simulink model "mathematical_inverted_pendulum_2018"  (R2018a)
settings: Solver=ode5  StartTime=0.0  StopTime=2  FixedStep=10e-6  RelTol=1e-3
values from neighbouring files (symbols this model uses):
  b = 0.1    [inverted_pendulum_parameter.m]
  g = 9.8    [inverted_pendulum_parameter.m]
  I = 0.006    [inverted_pendulum_parameter.m]
  l = 0.3    [inverted_pendulum_parameter.m]
  M = 0.5    [inverted_pendulum_parameter.m]
  m = 0.2    [inverted_pendulum_parameter.m]
settings Model: Creator=Goku  LastModifiedBy=root
settings DataIOCC: ReturnWorkspaceOutputs=on
settings DebuggingCC: InitInArrayFormatMsg=none
settings SFSimCC: SimUseLocalCustomCode=on
settings RTWCC: RTWUseLocalCustomCode=on

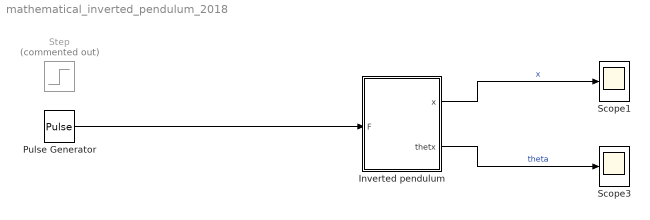
== system mathematical_inverted_pendulum_2018 ==
  Inverted pendulum : Subsystem
  Pulse Generator : DiscretePulseGenerator  PulseType=Time based  Amplitude=1000  Period=10  PulseWidth=0.01
  Scope1 : Scope
  Scope3 : Scope
  Step : Step  Commented=on  Time=0.01  Before=1  After=0  SampleTime=0
  wires:
  Inverted pendulum/1(x) -> Scope1/1  "x"
  Inverted pendulum/2(thetx) -> Scope3/1  "theta"
  Pulse Generator/1 -> Inverted pendulum/1(F)

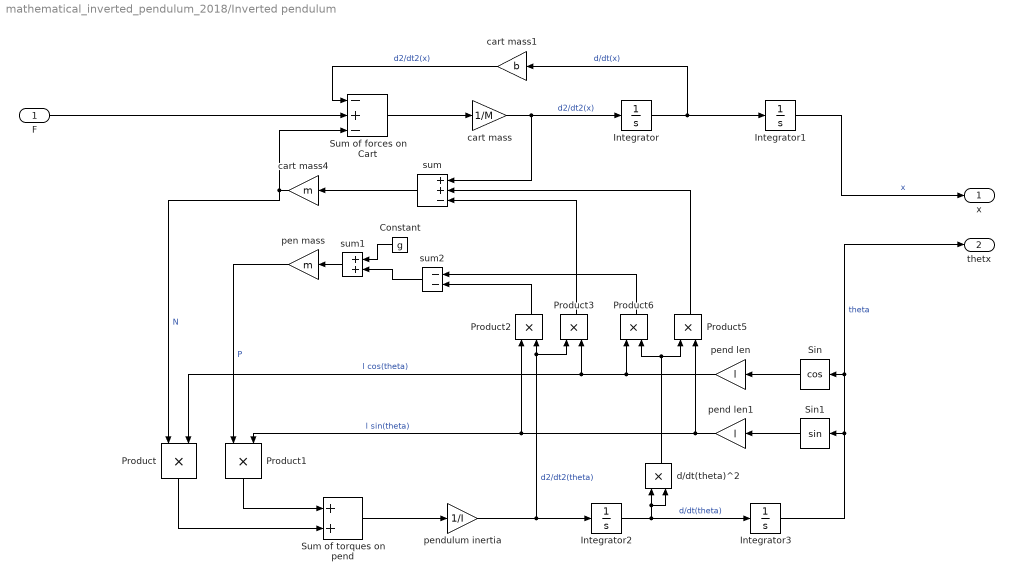
== system mathematical_inverted_pendulum_2018/Inverted pendulum ==
  F : Inport
  Constant : Constant  Value=g
  Integrator{,1..3} (4 alike) : Integrator
  Product{,1..3,5..6} (6 alike) : Product
  Sin : Trigonometry  Operator=cos
  Sin1 : Trigonometry
  Sum of forces on Cart : Sum  Inputs=-+-
  Sum of torques on pend : Sum
  cart mass : Gain  Gain=1/M
  cart mass1 : Gain  Gain=b
  cart mass4 : Gain  Gain=m
  d/dt(theta)^2 : Product
  pen mass : Gain  Gain=m
  pend len : Gain  Gain=l
  pend len1 : Gain  Gain=l
  pendulum inertia : Gain  Gain=1/I
  sum : Sum  Inputs=++-
  sum1 : Sum
  sum2 : Sum  Inputs=--
  x : Outport  VectorParamsAs1DForOutWhenUnconnected=on
  thetx : Outport  Port=2  VectorParamsAs1DForOutWhenUnconnected=on
  wires:
  Sum of forces on Cart/1 -> cart mass/1
  Integrator/1 -> cart mass1/1, Integrator1/1  "d/dt(x)"
  Product1/1 -> Sum of torques on pend/1
  Constant/1 -> sum1/1
  Integrator3/1 -> thetx/1, Sin/1, Sin1/1  "theta"
  pen mass/1 -> Product1/1  "P"
  Product3/1 -> sum/3
  Integrator1/1 -> x/1  "x"
  cart mass1/1 -> Sum of forces on Cart/1  "d2/dt2(x)"
  Sin/1 -> pend len/1
  sum2/1 -> sum1/2
  cart mass4/1 -> Product/1, Sum of forces on Cart/3  "N"
  cart mass/1 -> sum/1, Integrator/1  "d2/dt2(x)"
  Sum of torques on pend/1 -> pendulum inertia/1
  Product6/1 -> sum2/1
  pendulum inertia/1 -> Product3/1, Product2/2, Integrator2/1  "d2/dt2(theta)"
  Product/1 -> Sum of torques on pend/2
  F/1 -> Sum of forces on Cart/2
  pend len/1 -> Product6/1, Product3/2, Product/2  "l cos(theta)"
  sum1/1 -> pen mass/1
  Sin1/1 -> pend len1/1
  Product2/1 -> sum2/2
  d/dt(theta)^2/1 -> Product5/1, Product6/2
  sum/1 -> cart mass4/1
  pend len1/1 -> Product2/1, Product1/2, Product5/2  "l sin(theta)"
  Product5/1 -> sum/2
  Integrator2/1 -> Integrator3/1, d/dt(theta)^2/2, d/dt(theta)^2/1  "d/dt(theta)"
